simulink model "example2_IAM_b0"  (R2013b)
settings: Solver=ode45  StartTime=0  StopTime=24*3600  RelTol=1e-3
libraries: carnot x2
settings Model: Creator=drhf  LastModifiedBy=drhf
settings OptimizationCC: ExpressionDepthLimit=2147483647
settings DebuggingCC: StateNameClashWarn=warning
settings GRTTargetCC: CombineOutputUpdateFcns=off  GRTInterface=on

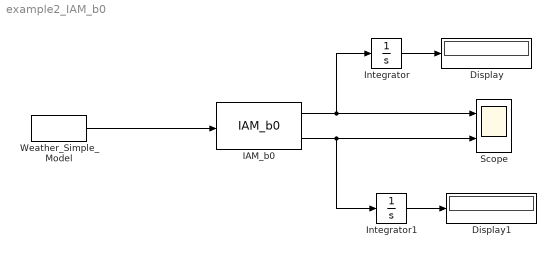
== system example2_IAM_b0 ==
  Display : Display
  Display1 : Display
  IAM_b0 : carnot/Source/Solar_Thermal/IncidenceAngleModifier/IAM_b0  b0=0.12  Kd=0.92  fta=1
  Integrator : Integrator
  Integrator1 : Integrator
  Scope : Scope  NumInputPorts=2
      settings: YMin=-5~-5  YMax=5~5
  Weather_Simple_Model : carnot/Weather/Weather_Simple_Model  lat=0  Ibn=900  Idg=100  tamb=5  deltaTsky=-6  rh=50  precip="10e-3/24/3600           % 10 mm in 24 h"  cloud=0.125  p=1013e2  vw=1  wdir=270
  wires:
  IAM_b0/1 -> Scope/1, Integrator/1
  IAM_b0/2 -> Scope/2, Integrator1/1
  Integrator/1 -> Display/1
  Weather_Simple_Model/1 -> IAM_b0/1
  Integrator1/1 -> Display1/1
